simulink model "untitled"  (R2025b)
settings: Solver=VariableStepAuto  StartTime=0.0  StopTime=10.0  RelTol=1e-3
libraries: mcbplantlib x4, autolibbldc x4, mcbhdlpositiondecoderlib x4, slpidlib x1
settings Model: Creator=JEDIDAH  LastModifiedBy=JEDIDAH

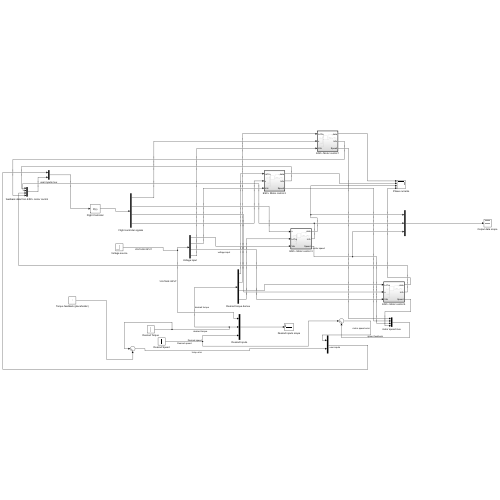
[thumbnail: Simulink's stored preview of the top-level diagram]
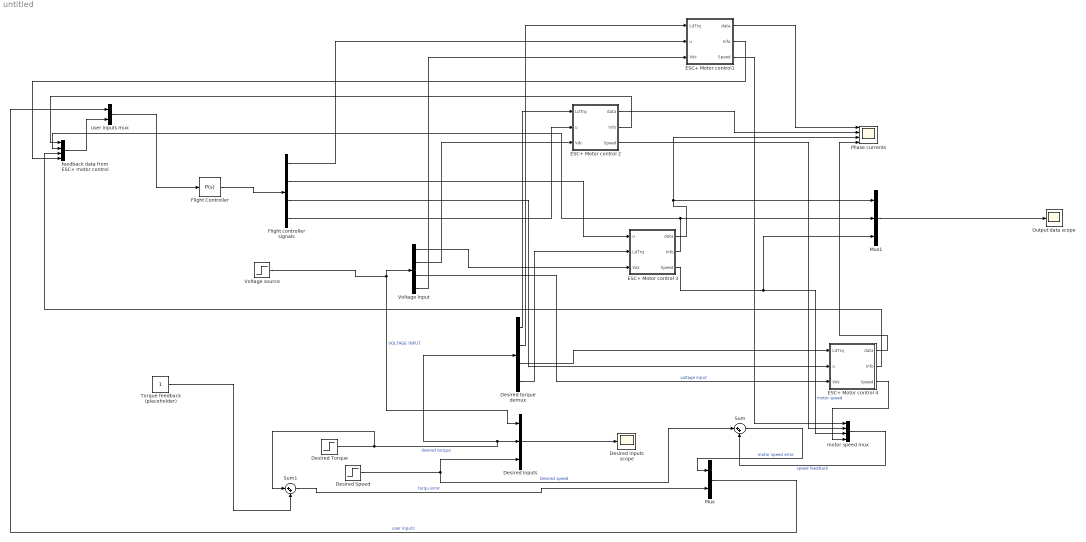
== system untitled ==
  Desired Inputs : Mux  Inputs=3
  Desired Speed : Step  SampleTime=0
  Desired Torque : Step  SampleTime=0
  Desired inputs scope : Scope
      settings: DataLoggingVariableName=ScopeData2
  Desired torque demux : Demux
  ESC+ Motor control 2 : Subsystem  TreatAsAtomicUnit=on
  ESC+ Motor control 3 : Subsystem  TreatAsAtomicUnit=on
  ESC+ Motor control 4 : Subsystem  TreatAsAtomicUnit=on
  ESC+ Motor control1 : Subsystem  TreatAsAtomicUnit=on
  Flight Controller : slpidlib/PID Controller  Controller=P  Form=Parallel  TimeDomain=Continuous-time  UseExternalTs=off  SampleTime=-1  IntegratorMethod=Forward Euler  FilterMethod=Forward Euler  ControllerParametersSource=internal  P=1  I=1  UseKiTs=off  D=0  UseExternalDerivativeSource=off  N=100  UseFilter=on  TunerSelectOption=Transfer Function Based (PID Tuner App)  InitialConditionSource=internal  InitialConditionForIntegrator=0  InitialConditionForFilter=0  DifferentiatorICPrevScaledInput=0  ExternalReset=none  TrackingMode=off  Kt=1  LimitOutput=off  SatLimitsSource=internal  UpperSaturationLimit=inf  LowerSaturationLimit=-inf  LinearizeAsGain=on  AntiWindupMode=none  Kb=1  LimitIntegrator=off  UpperIntegratorSaturationLimit=inf  LowerIntegratorSaturationLimit=-inf  POutMin=[]  POutMax=[]  IOutMin=[]  IOutMax=[]  DOutMin=[]  DOutMax=[]  NOutMin=[]  NOutMax=[]  SumOutMin=[]  SumOutMax=[]  SaturationOutMin=[]  SaturationOutMax=[]  PParamMin=[]  PParamMax=[]  IParamMin=[]  IParamMax=[]  DParamMin=[]  DParamMax=[]  NParamMin=[]  NParamMax=[]  KbParamMin=[]  KbParamMax=[]  KtParamMin=[]  KtParamMax=[]  KbOutMin=[]  KbOutMax=[]  KtOutMin=[]  KtOutMax=[]  IntegratorOutMin=[]  IntegratorOutMax=[]  FilterOutMin=[]  FilterOutMax=[]  SumI1OutMin=[]  SumI1OutMax=[]  SumI2OutMin=[]  SumI2OutMax=[]  SumI3OutMin=[]  SumI3OutMax=[]  SumI4OutMin=[]  SumI4OutMax=[]  SumDOutMin=[]  SumDOutMax=[]  DifferentiatorOutMin=[]  DifferentiatorOutMax=[]  FilterDiffOutCoefMin=[]  FilterDiffOutCoefMax=[]  ReciprocalOutMin=[]  ReciprocalOutMax=[]  SumDenOutMin=[]  SumDenOutMax=[]  SumNumOutMin=[]  SumNumOutMax=[]  DivideOutMin=[]  DivideOutMax=[]  UdiffTsProdOutMin=[]  UdiffTsProdOutMax=[]  NTsProdOutMin=[]  NTsProdOutMax=[]  UintegralTsProdOutMin=[]  UintegralTsProdOutMax=[]  UngainTsProdOutMin=[]  UngainTsProdOutMax=[]  ClampingZeroOutDataTypeStr=Inherit: Inherit via back propagation  ClampingZeroOutMin=[]  ClampingZeroOutMax=[]  FilterDenConstantOutDataTypeStr=Inherit: Inherit via back propagation  FilterDenConstantOutMin=[]  FilterDenConstantOutMax=[]  PCopyOutDataTypeStr=Inherit: Inherit via back propagation  PCopyOutMin=[]  PCopyOutMax=[]  NCopyOutDataTypeStr=Inherit: Inherit via back propagation  NCopyOutMin=[]  NCopyOutMax=[]  IntegratorContinuousStateAttributes=''  IntegratorStateMustResolveToSignalObject=off  IntegratorRTWStateStorageClass=Auto  FilterContinuousStateAttributes=''  FilterStateMustResolveToSignalObject=off  FilterRTWStateStorageClass=Auto  ParallelPVariant=InternalParameters  IdealPVariant=Disabled  IVariant=Disabled  DVariant=Disabled  IntegratorVariant=Disabled  SatVariant=Disabled  AWVariant=Disabled  PCopyVariant=Disabled  TRVariant=Disabled  FdbkBlocksVariant=Forward  IdealPFdbkVariant=Disabled  SatFdbkVariant=Disabled  DerivativeFilterVariant=Disabled  NVariant=Disabled  NCopyVariant=Disabled_SignalSpec  FilterICVariant=Disabled  IntegratorICVariant=Disabled  ExternalResetVariant=Disabled  TRSumVariant=Passthrough  SumFdbkVariant=Disabled  SumVariant=Passthrough_P  TsampFilterVariant=InternalTs  TsampNgainVariant=Passthrough  TsampIntegralVariant=Disabled_SignalSpec  ExternalSaturationOutDataTypeStr=Inherit: Same as second input  DerivativeSourceVariant=Disabled  PreIntVariant=InternalPreInt
  Flight controller signals : Demux
  Mux : Mux  Inputs=2
  Mux1 : Mux  Inputs=3
  Output data scope : Scope
  Phase currents : Scope  NumInputPorts=4
  Sum : Sum  Inputs=|++
  Sum1 : Sum  Inputs=|++
  Torque feedback (placeholder) : Constant
  Voltage input : Demux
  Voltage source : Step  SampleTime=0
  feedback data from ESC+ motor control : Mux
  motor speed mux : Mux
  user inputs mux : Mux  Inputs=2
  wires:
  Desired Speed/1 -> Desired Inputs/3, Sum/1  "Desired speed"
  Desired Torque/1 -> Sum1/1, Desired torque demux/1, Desired Inputs/2  "desired torque"
  Flight Controller/1 -> Flight controller signals/1
  Voltage source/1 -> Desired Inputs/1, Voltage input/1  "VOLTAGE INPUT"
  Flight controller signals/1 -> ESC+ Motor control1/2(u)
  Flight controller signals/2 -> ESC+ Motor control 3/1(u)
  Flight controller signals/3 -> ESC+ Motor control 4/2(u)
  ESC+ Motor control 3/3(Speed) -> motor speed mux/3, Mux1/3  "motor speed"
  Flight controller signals/4 -> ESC+ Motor control 2/2(u)
  Voltage input/4 -> ESC+ Motor control1/3(Vdc)
  Voltage input/3 -> ESC+ Motor control 4/3(Vdc)  "voltage input"
  Voltage input/2 -> ESC+ Motor control 2/3(Vdc)
  Voltage input/1 -> ESC+ Motor control 3/3(Vdc)
  Desired torque demux/2 -> ESC+ Motor control1/1(LdTrq)
  Desired torque demux/1 -> ESC+ Motor control 2/1(LdTrq)
  Desired torque demux/3 -> ESC+ Motor control 4/1(LdTrq)
  Desired torque demux/4 -> ESC+ Motor control 3/2(LdTrq)
  Desired Inputs/1 -> Desired inputs scope/1
  ESC+ Motor control 3/1(data) -> Mux1/1, Phase currents/3
  ESC+ Motor control 3/2(Info) -> feedback data from ESC+ motor control/2, Mux1/2
  Sum/1 -> Mux/1  "motor speed error"
  Mux1/1 -> Output data scope/1
  ESC+ Motor control 2/1(data) -> Phase currents/2
  ESC+ Motor control1/1(data) -> Phase currents/1
  ESC+ Motor control 4/1(data) -> Phase currents/4
  user inputs mux/1 -> Flight Controller/1
  ESC+ Motor control 4/2(Info) -> feedback data from ESC+ motor control/3
  ESC+ Motor control1/2(Info) -> feedback data from ESC+ motor control/4
  ESC+ Motor control 2/2(Info) -> feedback data from ESC+ motor control/1
  feedback data from ESC+ motor control/1 -> user inputs mux/2
  Torque feedback (placeholder)/1 -> Sum1/2
  Sum1/1 -> Mux/2  "torqu error"
  motor speed mux/1 -> Sum/2  "speed feedback"
  ESC+ Motor control 4/3(Speed) -> motor speed mux/4
  ESC+ Motor control 2/3(Speed) -> motor speed mux/2
  ESC+ Motor control1/3(Speed) -> motor speed mux/1
  Mux/1 -> user inputs mux/1  "user inputs"

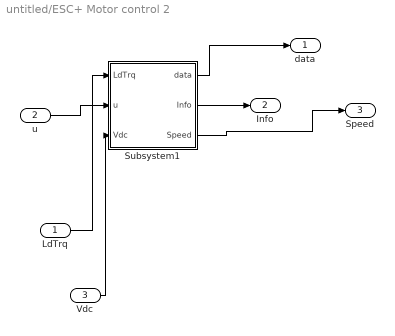
== system untitled/ESC+ Motor control 2 ==
  LdTrq : Inport
  u : Inport  Port=2
  Vdc : Inport  Port=3
  Subsystem1 : Subsystem  TreatAsAtomicUnit=on
  data : Outport
  Info : Outport  Port=2
  Speed : Outport  Port=3
  wires:
  Subsystem1/1(data) -> data/1
  Vdc/1 -> Subsystem1/3(Vdc)
  LdTrq/1 -> Subsystem1/1(LdTrq)
  u/1 -> Subsystem1/2(u)
  Subsystem1/2(Info) -> Info/1
  Subsystem1/3(Speed) -> Speed/1

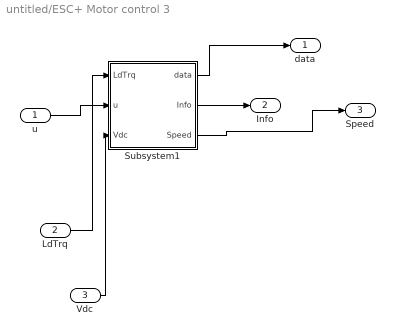
== system untitled/ESC+ Motor control 3 ==
  u : Inport
  LdTrq : Inport  Port=2
  Vdc : Inport  Port=3
  Subsystem1 : Subsystem  TreatAsAtomicUnit=on
  data : Outport
  Info : Outport  Port=2
  Speed : Outport  Port=3
  wires:
  Subsystem1/1(data) -> data/1
  Vdc/1 -> Subsystem1/3(Vdc)
  LdTrq/1 -> Subsystem1/1(LdTrq)
  u/1 -> Subsystem1/2(u)
  Subsystem1/2(Info) -> Info/1
  Subsystem1/3(Speed) -> Speed/1

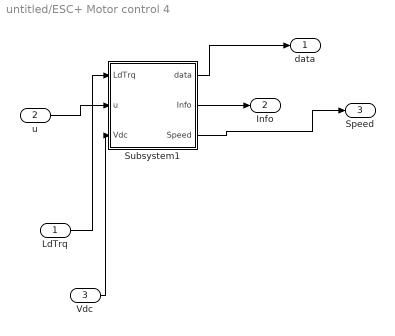
== system untitled/ESC+ Motor control 4 ==
  LdTrq : Inport
  u : Inport  Port=2
  Vdc : Inport  Port=3
  Subsystem1 : Subsystem  TreatAsAtomicUnit=on
  data : Outport
  Info : Outport  Port=2
  Speed : Outport  Port=3
  wires:
  Subsystem1/1(data) -> data/1
  Vdc/1 -> Subsystem1/3(Vdc)
  LdTrq/1 -> Subsystem1/1(LdTrq)
  u/1 -> Subsystem1/2(u)
  Subsystem1/2(Info) -> Info/1
  Subsystem1/3(Speed) -> Speed/1

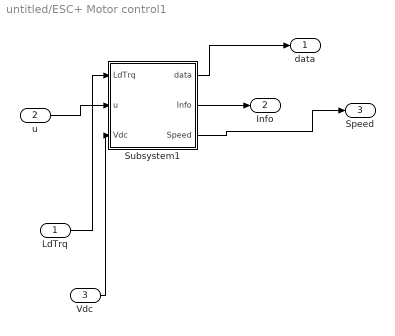
== system untitled/ESC+ Motor control1 ==
  LdTrq : Inport
  u : Inport  Port=2
  Vdc : Inport  Port=3
  Subsystem1 : Subsystem  TreatAsAtomicUnit=on
  data : Outport
  Info : Outport  Port=2
  Speed : Outport  Port=3
  wires:
  Subsystem1/1(data) -> data/1
  Vdc/1 -> Subsystem1/3(Vdc)
  LdTrq/1 -> Subsystem1/1(LdTrq)
  u/1 -> Subsystem1/2(u)
  Subsystem1/2(Info) -> Info/1
  Subsystem1/3(Speed) -> Speed/1

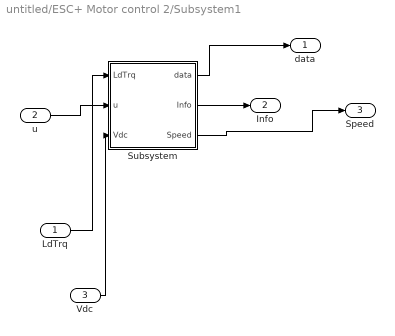
== system untitled/ESC+ Motor control 2/Subsystem1 ==
  LdTrq : Inport
  u : Inport  Port=2
  Vdc : Inport  Port=3
  Subsystem : Subsystem  TreatAsAtomicUnit=on
  data : Outport
  Info : Outport  Port=2
  Speed : Outport  Port=3
  wires:
  Subsystem/1(data) -> data/1
  Vdc/1 -> Subsystem/3(Vdc)
  LdTrq/1 -> Subsystem/1(LdTrq)
  Subsystem/2(Info) -> Info/1
  u/1 -> Subsystem/2(u)
  Subsystem/3(Speed) -> Speed/1

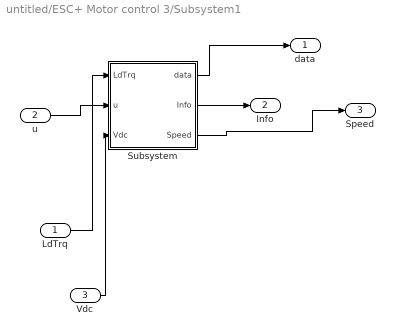
== system untitled/ESC+ Motor control 3/Subsystem1 ==
  LdTrq : Inport
  u : Inport  Port=2
  Vdc : Inport  Port=3
  Subsystem : Subsystem  TreatAsAtomicUnit=on
  data : Outport
  Info : Outport  Port=2
  Speed : Outport  Port=3
  wires:
  Subsystem/1(data) -> data/1
  Vdc/1 -> Subsystem/3(Vdc)
  LdTrq/1 -> Subsystem/1(LdTrq)
  Subsystem/2(Info) -> Info/1
  u/1 -> Subsystem/2(u)
  Subsystem/3(Speed) -> Speed/1

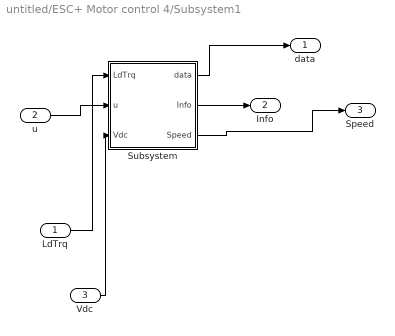
== system untitled/ESC+ Motor control 4/Subsystem1 ==
  LdTrq : Inport
  u : Inport  Port=2
  Vdc : Inport  Port=3
  Subsystem : Subsystem  TreatAsAtomicUnit=on
  data : Outport
  Info : Outport  Port=2
  Speed : Outport  Port=3
  wires:
  Subsystem/1(data) -> data/1
  Vdc/1 -> Subsystem/3(Vdc)
  LdTrq/1 -> Subsystem/1(LdTrq)
  Subsystem/2(Info) -> Info/1
  u/1 -> Subsystem/2(u)
  Subsystem/3(Speed) -> Speed/1

== system untitled/ESC+ Motor control1/Subsystem1 ==
  LdTrq : Inport
  u : Inport  Port=2
  Vdc : Inport  Port=3
  Subsystem : Subsystem  TreatAsAtomicUnit=on
  data : Outport
  Info : Outport  Port=2
  Speed : Outport  Port=3
  wires:
  Subsystem/1(data) -> data/1
  Vdc/1 -> Subsystem/3(Vdc)
  LdTrq/1 -> Subsystem/1(LdTrq)
  Subsystem/2(Info) -> Info/1
  u/1 -> Subsystem/2(u)
  Subsystem/3(Speed) -> Speed/1

== system untitled/ESC+ Motor control 2/Subsystem1/Subsystem ==
  LdTrq : Inport
  u : Inport  Port=2
  Vdc : Inport  Port=3
  Subsystem1 : Subsystem  TreatAsAtomicUnit=on
  data : Outport
  Info : Outport  Port=2
  Speed : Outport  Port=3
  wires:
  LdTrq/1 -> Subsystem1/1(LdTrq)
  Subsystem1/2(Info) -> Info/1
  u/1 -> Subsystem1/2(u)
  Subsystem1/3(Speed) -> Speed/1
  Subsystem1/1(data) -> data/1
  Vdc/1 -> Subsystem1/3(Vdc)

== system untitled/ESC+ Motor control 3/Subsystem1/Subsystem ==
  LdTrq : Inport
  u : Inport  Port=2
  Vdc : Inport  Port=3
  Subsystem1 : Subsystem  TreatAsAtomicUnit=on
  data : Outport
  Info : Outport  Port=2
  Speed : Outport  Port=3
  wires:
  LdTrq/1 -> Subsystem1/1(LdTrq)
  Subsystem1/2(Info) -> Info/1
  u/1 -> Subsystem1/2(u)
  Subsystem1/3(Speed) -> Speed/1
  Subsystem1/1(data) -> data/1
  Vdc/1 -> Subsystem1/3(Vdc)

== system untitled/ESC+ Motor control 4/Subsystem1/Subsystem ==
  LdTrq : Inport
  u : Inport  Port=2
  Vdc : Inport  Port=3
  Subsystem1 : Subsystem  TreatAsAtomicUnit=on
  data : Outport
  Info : Outport  Port=2
  Speed : Outport  Port=3
  wires:
  LdTrq/1 -> Subsystem1/1(LdTrq)
  Subsystem1/2(Info) -> Info/1
  u/1 -> Subsystem1/2(u)
  Subsystem1/3(Speed) -> Speed/1
  Subsystem1/1(data) -> data/1
  Vdc/1 -> Subsystem1/3(Vdc)

== system untitled/ESC+ Motor control1/Subsystem1/Subsystem ==
  LdTrq : Inport
  u : Inport  Port=2
  Vdc : Inport  Port=3
  Subsystem1 : Subsystem  TreatAsAtomicUnit=on
  data : Outport
  Info : Outport  Port=2
  Speed : Outport  Port=3
  wires:
  LdTrq/1 -> Subsystem1/1(LdTrq)
  Subsystem1/2(Info) -> Info/1
  u/1 -> Subsystem1/2(u)
  Subsystem1/3(Speed) -> Speed/1
  Subsystem1/1(data) -> data/1
  Vdc/1 -> Subsystem1/3(Vdc)

== system untitled/ESC+ Motor control 2/Subsystem1/Subsystem/Subsystem1 ==
  LdTrq : Inport
  u : Inport  Port=2
  Vdc : Inport  Port=3
  Subsystem : Subsystem  TreatAsAtomicUnit=on
  data : Outport
  Info : Outport  Port=2
  Speed : Outport  Port=3
  wires:
  u/1 -> Subsystem/2(u)
  Subsystem/3(Speed) -> Speed/1
  Subsystem/1(data) -> data/1
  Subsystem/2(Info) -> Info/1
  LdTrq/1 -> Subsystem/1(LdTrq)
  Vdc/1 -> Subsystem/3(Vdc)

== system untitled/ESC+ Motor control 3/Subsystem1/Subsystem/Subsystem1 ==
  LdTrq : Inport
  u : Inport  Port=2
  Vdc : Inport  Port=3
  Subsystem : Subsystem  TreatAsAtomicUnit=on
  data : Outport
  Info : Outport  Port=2
  Speed : Outport  Port=3
  wires:
  u/1 -> Subsystem/2(u)
  Subsystem/3(Speed) -> Speed/1
  Subsystem/1(data) -> data/1
  Subsystem/2(Info) -> Info/1
  LdTrq/1 -> Subsystem/1(LdTrq)
  Vdc/1 -> Subsystem/3(Vdc)

== system untitled/ESC+ Motor control 4/Subsystem1/Subsystem/Subsystem1 ==
  LdTrq : Inport
  u : Inport  Port=2
  Vdc : Inport  Port=3
  Subsystem : Subsystem  TreatAsAtomicUnit=on
  data : Outport
  Info : Outport  Port=2
  Speed : Outport  Port=3
  wires:
  u/1 -> Subsystem/2(u)
  Subsystem/3(Speed) -> Speed/1
  Subsystem/1(data) -> data/1
  Subsystem/2(Info) -> Info/1
  LdTrq/1 -> Subsystem/1(LdTrq)
  Vdc/1 -> Subsystem/3(Vdc)

== system untitled/ESC+ Motor control1/Subsystem1/Subsystem/Subsystem1 ==
  LdTrq : Inport
  u : Inport  Port=2
  Vdc : Inport  Port=3
  Subsystem : Subsystem  TreatAsAtomicUnit=on
  data : Outport
  Info : Outport  Port=2
  Speed : Outport  Port=3
  wires:
  u/1 -> Subsystem/2(u)
  Subsystem/3(Speed) -> Speed/1
  Subsystem/1(data) -> data/1
  Subsystem/2(Info) -> Info/1
  LdTrq/1 -> Subsystem/1(LdTrq)
  Vdc/1 -> Subsystem/3(Vdc)

== system untitled/ESC+ Motor control 2/Subsystem1/Subsystem/Subsystem1/Subsystem ==
  LdTrq : Inport
  u : Inport  Port=2
  Vdc : Inport  Port=3
  Subsystem1 : Subsystem  TreatAsAtomicUnit=on
  data : Outport
  Info : Outport  Port=2
  Speed : Outport  Port=3
  wires:
  Subsystem1/3(Speed) -> Speed/1
  Subsystem1/1(data) -> data/1
  u/1 -> Subsystem1/2(u)
  LdTrq/1 -> Subsystem1/1(LdTrq)
  Subsystem1/2(Info) -> Info/1
  Vdc/1 -> Subsystem1/3(Vdc)

== system untitled/ESC+ Motor control 3/Subsystem1/Subsystem/Subsystem1/Subsystem ==
  LdTrq : Inport
  u : Inport  Port=2
  Vdc : Inport  Port=3
  Subsystem1 : Subsystem  TreatAsAtomicUnit=on
  data : Outport
  Info : Outport  Port=2
  Speed : Outport  Port=3
  wires:
  Subsystem1/3(Speed) -> Speed/1
  Subsystem1/1(data) -> data/1
  u/1 -> Subsystem1/2(u)
  LdTrq/1 -> Subsystem1/1(LdTrq)
  Subsystem1/2(Info) -> Info/1
  Vdc/1 -> Subsystem1/3(Vdc)

== system untitled/ESC+ Motor control 4/Subsystem1/Subsystem/Subsystem1/Subsystem ==
  LdTrq : Inport
  u : Inport  Port=2
  Vdc : Inport  Port=3
  Subsystem1 : Subsystem  TreatAsAtomicUnit=on
  data : Outport
  Info : Outport  Port=2
  Speed : Outport  Port=3
  wires:
  Subsystem1/3(Speed) -> Speed/1
  Subsystem1/1(data) -> data/1
  u/1 -> Subsystem1/2(u)
  LdTrq/1 -> Subsystem1/1(LdTrq)
  Subsystem1/2(Info) -> Info/1
  Vdc/1 -> Subsystem1/3(Vdc)

== system untitled/ESC+ Motor control1/Subsystem1/Subsystem/Subsystem1/Subsystem ==
  LdTrq : Inport
  u : Inport  Port=2
  Vdc : Inport  Port=3
  Subsystem1 : Subsystem  TreatAsAtomicUnit=on
  data : Outport
  Info : Outport  Port=2
  Speed : Outport  Port=3
  wires:
  Subsystem1/3(Speed) -> Speed/1
  Subsystem1/1(data) -> data/1
  u/1 -> Subsystem1/2(u)
  LdTrq/1 -> Subsystem1/1(LdTrq)
  Subsystem1/2(Info) -> Info/1
  Vdc/1 -> Subsystem1/3(Vdc)

== system untitled/ESC+ Motor control 2/Subsystem1/Subsystem/Subsystem1/Subsystem/Subsystem1 ==
  LdTrq : Inport
  u : Inport  Port=2
  Vdc : Inport  Port=3
  Subsystem : Subsystem
  data : Outport
  Info : Outport  Port=2
  Speed : Outport  Port=3
  wires:
  Subsystem/1(PhCurr) -> data/1, Subsystem/2(data)
  LdTrq/1 -> Subsystem/1(LdTrq)
  u/1 -> Subsystem/3(u)
  Subsystem/2(Info) -> Info/1
  Subsystem/3(Speed) -> Speed/1
  Vdc/1 -> Subsystem/4(Vdc)

== system untitled/ESC+ Motor control 3/Subsystem1/Subsystem/Subsystem1/Subsystem/Subsystem1 ==
  LdTrq : Inport
  u : Inport  Port=2
  Vdc : Inport  Port=3
  Subsystem : Subsystem
  data : Outport
  Info : Outport  Port=2
  Speed : Outport  Port=3
  wires:
  Subsystem/1(PhCurr) -> data/1, Subsystem/2(data)
  LdTrq/1 -> Subsystem/1(LdTrq)
  u/1 -> Subsystem/3(u)
  Subsystem/2(Info) -> Info/1
  Subsystem/3(Speed) -> Speed/1
  Vdc/1 -> Subsystem/4(Vdc)

== system untitled/ESC+ Motor control 4/Subsystem1/Subsystem/Subsystem1/Subsystem/Subsystem1 ==
  LdTrq : Inport
  u : Inport  Port=2
  Vdc : Inport  Port=3
  Subsystem : Subsystem
  data : Outport
  Info : Outport  Port=2
  Speed : Outport  Port=3
  wires:
  Subsystem/1(PhCurr) -> data/1, Subsystem/2(data)
  LdTrq/1 -> Subsystem/1(LdTrq)
  u/1 -> Subsystem/3(u)
  Subsystem/2(Info) -> Info/1
  Subsystem/3(Speed) -> Speed/1
  Vdc/1 -> Subsystem/4(Vdc)

== system untitled/ESC+ Motor control1/Subsystem1/Subsystem/Subsystem1/Subsystem/Subsystem1 ==
  LdTrq : Inport
  u : Inport  Port=2
  Vdc : Inport  Port=3
  Subsystem : Subsystem
  data : Outport
  Info : Outport  Port=2
  Speed : Outport  Port=3
  wires:
  Subsystem/1(PhCurr) -> data/1, Subsystem/2(data)
  LdTrq/1 -> Subsystem/1(LdTrq)
  u/1 -> Subsystem/3(u)
  Subsystem/2(Info) -> Info/1
  Subsystem/3(Speed) -> Speed/1
  Vdc/1 -> Subsystem/4(Vdc)

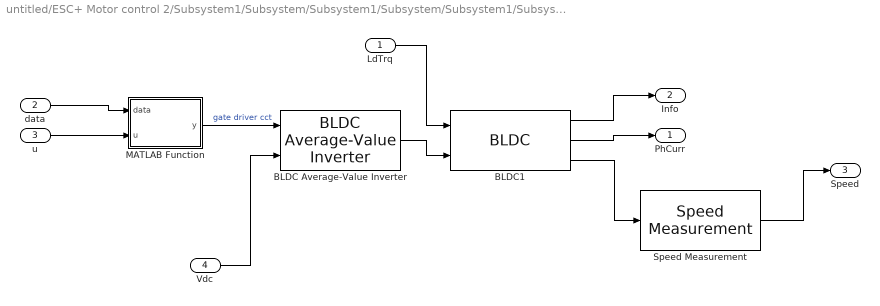
== system untitled/ESC+ Motor control 2/Subsystem1/Subsystem/Subsystem1/Subsystem/Subsystem1/Subsystem ==
  LdTrq : Inport
  data : Inport  Port=2
  u : Inport  Port=3
  Vdc : Inport  Port=4
  BLDC Average-Value Inverter : mcbplantlib/BLDC Average-Value Inverter
      settings: LibrarySourceBlock=mcblib/Electrical Systems/Inverters/BLDC Average-Value Inverter
  BLDC1 : autolibbldc/BLDC  VariantControl=pmsmVariant==pmsmEnum.TorqueInput  MechInput=Torque  SimType=Continuous  BlockSampleTime=25e-6  p=4  Rs=0.36  Ld=2e-4  Lq=2e-4  Lambda=0.0064  J=7.0616e-06  B=2.6369e-06  F=0  Id_init=0  Iq_init=0  Th_init=0  Omega_init=0  RefBlkName='autolibbldc/BLDC'  aMode=5
      settings: LibrarySourceBlock=mcblib/Electrical Systems/Motors/BLDC
  MATLAB Function : MATLAB Function  TreatAsAtomicUnit=on
  Speed Measurement : mcbhdlpositiondecoderlib/Speed Measurement  PositionUnit=Radians  PositionScalingDatatype=uint32  SpeedCalculationMode=Maximum application speed  SampleTimeAsync=100e-6  MaximumApplicationSpeed=1000  SpeedResolution=5e-6  DelayLength=299  MaximumMeasurableSpeed=1000  MeasurableSpeedResolution=4.6566e-07  SpeedUnit=RPM  PerUnitSpeed=1000  SpeedDataType=single
      settings: LibrarySourceBlock=mcbhdllib/Sensor Decoders/Speed Measurement
  PhCurr : Outport
  Info : Outport  Port=2
  Speed : Outport  Port=3
  wires:
  Vdc/1 -> BLDC Average-Value Inverter/2
  data/1 -> MATLAB Function/1(data)
  BLDC Average-Value Inverter/1 -> BLDC1/2
  BLDC1/2 -> PhCurr/1
  MATLAB Function/1(y) -> BLDC Average-Value Inverter/1  "gate driver cct"
  BLDC1/3 -> Speed Measurement/1
  LdTrq/1 -> BLDC1/1
  BLDC1/1 -> Info/1
  u/1 -> MATLAB Function/2(u)
  Speed Measurement/1 -> Speed/1

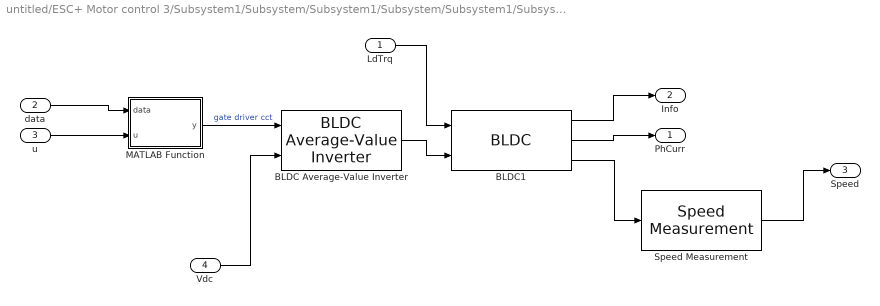
== system untitled/ESC+ Motor control 3/Subsystem1/Subsystem/Subsystem1/Subsystem/Subsystem1/Subsystem ==
  LdTrq : Inport
  data : Inport  Port=2
  u : Inport  Port=3
  Vdc : Inport  Port=4
  BLDC Average-Value Inverter : mcbplantlib/BLDC Average-Value Inverter
      settings: LibrarySourceBlock=mcblib/Electrical Systems/Inverters/BLDC Average-Value Inverter
  BLDC1 : autolibbldc/BLDC  VariantControl=pmsmVariant==pmsmEnum.TorqueInput  MechInput=Torque  SimType=Continuous  BlockSampleTime=25e-6  p=4  Rs=0.36  Ld=2e-4  Lq=2e-4  Lambda=0.0064  J=7.0616e-06  B=2.6369e-06  F=0  Id_init=0  Iq_init=0  Th_init=0  Omega_init=0  RefBlkName='autolibbldc/BLDC'  aMode=5
      settings: LibrarySourceBlock=mcblib/Electrical Systems/Motors/BLDC
  MATLAB Function : MATLAB Function  TreatAsAtomicUnit=on
  Speed Measurement : mcbhdlpositiondecoderlib/Speed Measurement  PositionUnit=Radians  PositionScalingDatatype=uint32  SpeedCalculationMode=Maximum application speed  SampleTimeAsync=100e-6  MaximumApplicationSpeed=1000  SpeedResolution=5e-6  DelayLength=299  MaximumMeasurableSpeed=1000  MeasurableSpeedResolution=4.6566e-07  SpeedUnit=RPM  PerUnitSpeed=1000  SpeedDataType=single
      settings: LibrarySourceBlock=mcbhdllib/Sensor Decoders/Speed Measurement
  PhCurr : Outport
  Info : Outport  Port=2
  Speed : Outport  Port=3
  wires:
  Vdc/1 -> BLDC Average-Value Inverter/2
  data/1 -> MATLAB Function/1(data)
  BLDC Average-Value Inverter/1 -> BLDC1/2
  BLDC1/2 -> PhCurr/1
  MATLAB Function/1(y) -> BLDC Average-Value Inverter/1  "gate driver cct"
  BLDC1/3 -> Speed Measurement/1
  LdTrq/1 -> BLDC1/1
  BLDC1/1 -> Info/1
  u/1 -> MATLAB Function/2(u)
  Speed Measurement/1 -> Speed/1

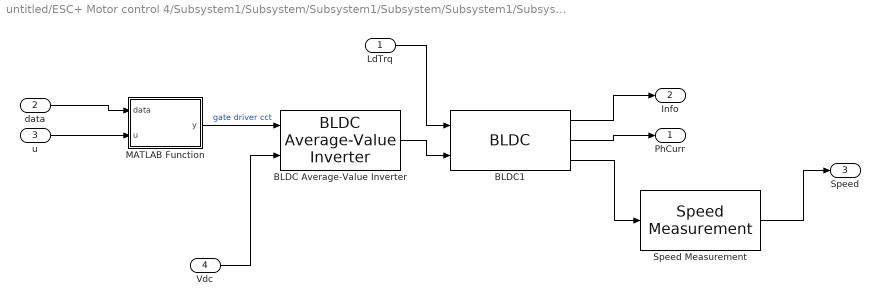
== system untitled/ESC+ Motor control 4/Subsystem1/Subsystem/Subsystem1/Subsystem/Subsystem1/Subsystem ==
  LdTrq : Inport
  data : Inport  Port=2
  u : Inport  Port=3
  Vdc : Inport  Port=4
  BLDC Average-Value Inverter : mcbplantlib/BLDC Average-Value Inverter
      settings: LibrarySourceBlock=mcblib/Electrical Systems/Inverters/BLDC Average-Value Inverter
  BLDC1 : autolibbldc/BLDC  VariantControl=pmsmVariant==pmsmEnum.TorqueInput  MechInput=Torque  SimType=Continuous  BlockSampleTime=25e-6  p=4  Rs=0.36  Ld=2e-4  Lq=2e-4  Lambda=0.0064  J=7.0616e-06  B=2.6369e-06  F=0  Id_init=0  Iq_init=0  Th_init=0  Omega_init=0  RefBlkName='autolibbldc/BLDC'  aMode=5
      settings: LibrarySourceBlock=mcblib/Electrical Systems/Motors/BLDC
  MATLAB Function : MATLAB Function  TreatAsAtomicUnit=on
  Speed Measurement : mcbhdlpositiondecoderlib/Speed Measurement  PositionUnit=Radians  PositionScalingDatatype=uint32  SpeedCalculationMode=Maximum application speed  SampleTimeAsync=100e-6  MaximumApplicationSpeed=1000  SpeedResolution=5e-6  DelayLength=299  MaximumMeasurableSpeed=1000  MeasurableSpeedResolution=4.6566e-07  SpeedUnit=RPM  PerUnitSpeed=1000  SpeedDataType=single
      settings: LibrarySourceBlock=mcbhdllib/Sensor Decoders/Speed Measurement
  PhCurr : Outport
  Info : Outport  Port=2
  Speed : Outport  Port=3
  wires:
  Vdc/1 -> BLDC Average-Value Inverter/2
  data/1 -> MATLAB Function/1(data)
  BLDC Average-Value Inverter/1 -> BLDC1/2
  BLDC1/2 -> PhCurr/1
  MATLAB Function/1(y) -> BLDC Average-Value Inverter/1  "gate driver cct"
  BLDC1/3 -> Speed Measurement/1
  LdTrq/1 -> BLDC1/1
  BLDC1/1 -> Info/1
  u/1 -> MATLAB Function/2(u)
  Speed Measurement/1 -> Speed/1

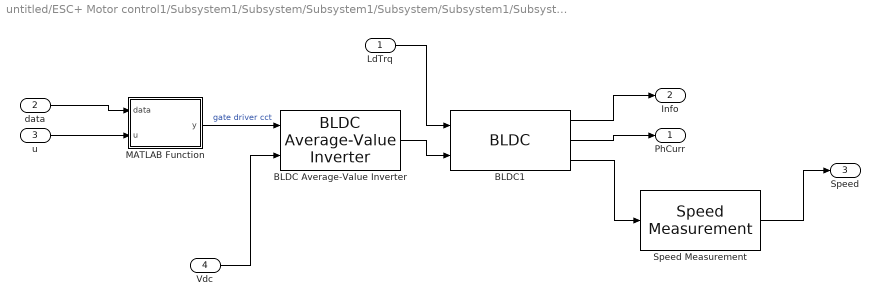
== system untitled/ESC+ Motor control1/Subsystem1/Subsystem/Subsystem1/Subsystem/Subsystem1/Subsystem ==
  LdTrq : Inport
  data : Inport  Port=2
  u : Inport  Port=3
  Vdc : Inport  Port=4
  BLDC Average-Value Inverter : mcbplantlib/BLDC Average-Value Inverter
      settings: LibrarySourceBlock=mcblib/Electrical Systems/Inverters/BLDC Average-Value Inverter
  BLDC1 : autolibbldc/BLDC  VariantControl=pmsmVariant==pmsmEnum.TorqueInput  MechInput=Torque  SimType=Continuous  BlockSampleTime=25e-6  p=4  Rs=0.36  Ld=2e-4  Lq=2e-4  Lambda=0.0064  J=7.0616e-06  B=2.6369e-06  F=0  Id_init=0  Iq_init=0  Th_init=0  Omega_init=0  RefBlkName='autolibbldc/BLDC'  aMode=5
      settings: LibrarySourceBlock=mcblib/Electrical Systems/Motors/BLDC
  MATLAB Function : MATLAB Function  TreatAsAtomicUnit=on
  Speed Measurement : mcbhdlpositiondecoderlib/Speed Measurement  PositionUnit=Radians  PositionScalingDatatype=uint32  SpeedCalculationMode=Maximum application speed  SampleTimeAsync=100e-6  MaximumApplicationSpeed=1000  SpeedResolution=5e-6  DelayLength=299  MaximumMeasurableSpeed=1000  MeasurableSpeedResolution=4.6566e-07  SpeedUnit=RPM  PerUnitSpeed=1000  SpeedDataType=single
      settings: LibrarySourceBlock=mcbhdllib/Sensor Decoders/Speed Measurement
  PhCurr : Outport
  Info : Outport  Port=2
  Speed : Outport  Port=3
  wires:
  Vdc/1 -> BLDC Average-Value Inverter/2
  data/1 -> MATLAB Function/1(data)
  BLDC Average-Value Inverter/1 -> BLDC1/2
  BLDC1/2 -> PhCurr/1
  MATLAB Function/1(y) -> BLDC Average-Value Inverter/1  "gate driver cct"
  BLDC1/3 -> Speed Measurement/1
  LdTrq/1 -> BLDC1/1
  BLDC1/1 -> Info/1
  u/1 -> MATLAB Function/2(u)
  Speed Measurement/1 -> Speed/1

== matlab function untitled/ESC+ Motor control 3/Subsystem1/Subsystem/Subsystem1/Subsystem/Subsystem1/Subsystem/MATLAB Function ==
  data: data input; u input; y output
function y = fcn(data, u)
%#codegen

y = u;

== matlab function untitled/ESC+ Motor control 4/Subsystem1/Subsystem/Subsystem1/Subsystem/Subsystem1/Subsystem/MATLAB Function ==
  data: data input; u input; y output
function y = fcn(data, u)
%#codegen

y = u;

== matlab function untitled/ESC+ Motor control 2/Subsystem1/Subsystem/Subsystem1/Subsystem/Subsystem1/Subsystem/MATLAB Function ==
  data: data input; u input; y output
function y = fcn(data, u)
%#codegen

y = u;

== matlab function untitled/ESC+ Motor control1/Subsystem1/Subsystem/Subsystem1/Subsystem/Subsystem1/Subsystem/MATLAB Function ==
  data: data input; u input; y output
function y = fcn(data, u)
%#codegen

y = u;
